simulink model "SimpleGyroModel"  (R2015b)
settings: Solver=ode5  StartTime=0.0  StopTime=180  FixedStep=1/819.2  RelTol=1e-3
values from neighbouring files (symbols this model uses):
  gyro_bias = 0.9140    (= 0.914)    [PrepCode.m]
  gyro_noise_density = 0.011    [PrepCode.m]
  gyro_sensitivity = 0.01    [PrepCode.m]    (also in Stm_constants.m = 0.7)
  w = lp_cutoff*2*pi    (= 2513.27412287)    [PrepCode.m]
  wn = gyroscope_wn    (= 17500)    [PrepCode.m]
  z = zeta    (= 0.5)    [PrepCode.m]    (also in Untitled5.m = [0 0 0 0 0 1;0 0 0 0 0 1;1 1 1 1 0 1;1 1 1 1 0 1]*s; drawCube.m = ([0 0 0 0 0 1;0 0 0 0 0 1;1 1 1 1 0 1;1 1 1 1 0 1]-0.5)*size)
  zeta = 0.5    [PrepCode.m]
libraries: simulink x2
settings Model: Creator=TOOsab  LastModifiedBy=TOOsab

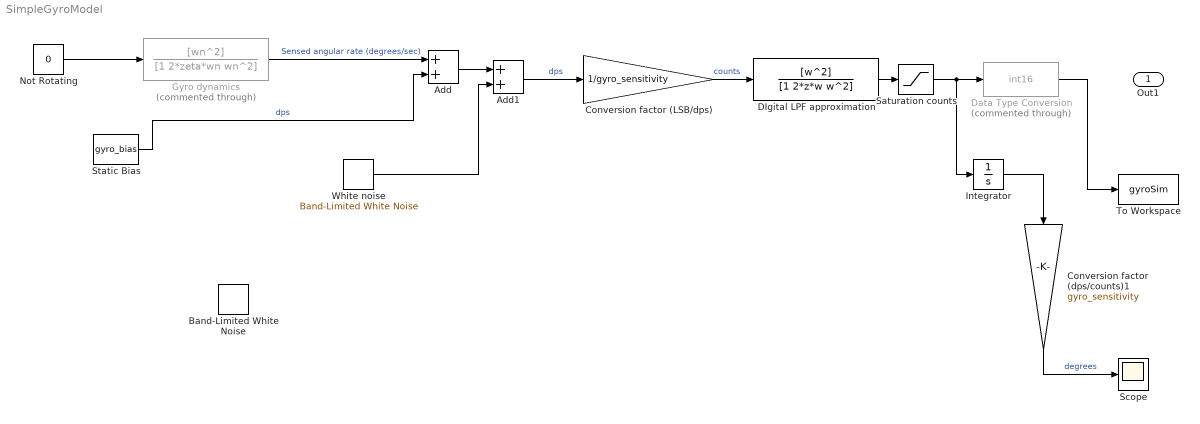
== system SimpleGyroModel ==
  Add : Sum
  Add1 : Sum
  Band-Limited White Noise : simulink/Sources/Band-Limited White Noise  Cov=[0.00247^2]  Ts=1/819.2  seed=[23341]
  Conversion factor (LSB/dps) : Gain  Gain=1/gyro_sensitivity
  Conversion factor (dps/counts)1 : Gain  Gain=gyro_sensitivity
  DIgital LPF approximation : TransferFcn  Numerator=[w^2]  Denominator=[1 2*z*w w^2]
  Data Type Conversion : DataTypeConversion  Commented=through  OutDataTypeStr=int16
  Gyro dynamics : TransferFcn  Commented=through  Numerator=[wn^2]  Denominator=[1 2*zeta*wn wn^2]
  Integrator : Integrator
  "Not Rotating " : Constant  Value=0
  "Saturation counts " : Saturate  UpperLimit=2^15  LowerLimit=-2^15
  Scope : Scope
  Static Bias : Constant  Value=gyro_bias
  To Workspace : ToWorkspace  VariableName=gyroSim  SampleTime=-1
  White noise : simulink/Sources/Band-Limited White Noise  Cov=[(gyro_noise_density/3)^2]  Ts=1/819.2  seed=[23341]
  Out1 : Outport
  wires:
  Conversion factor (LSB/dps)/1 -> DIgital LPF approximation/1  "counts"
  Static Bias/1 -> Add/2  "dps"
  Gyro dynamics/1 -> Add/1  "Sensed angular rate (degrees/sec)"
  White noise/1 -> Add1/2
  Add/1 -> Add1/1
  Add1/1 -> Conversion factor (LSB/dps)/1  "dps"
  DIgital LPF approximation/1 -> "Saturation counts "/1
  "Saturation counts "/1 -> Integrator/1, Data Type Conversion/1
  Data Type Conversion/1 -> To Workspace/1
  "Not Rotating "/1 -> Gyro dynamics/1
  Integrator/1 -> Conversion factor (dps/counts)1/1
  Conversion factor (dps/counts)1/1 -> Scope/1  "degrees"
